simulink model "vehicle_model"  (R2023a)
settings: configuration reference "SharedConfig" (kept outside this file)
undefined symbols (not defined in the file): config_vehicle
settings Model: Creator=frede  LastModifiedBy=polashehata
settings ConfigSetRef: SourceName=SharedConfig  SourceLocation=Base Workspace

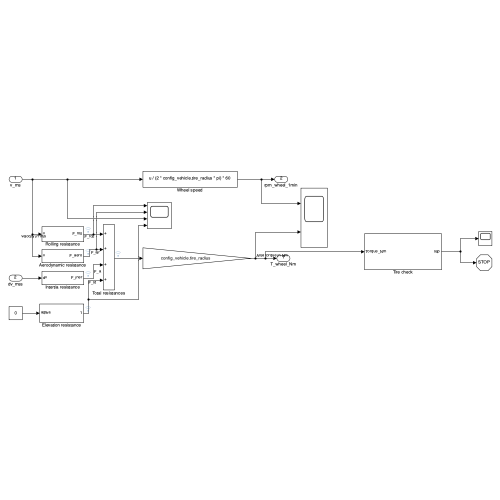
[thumbnail: Simulink's stored preview of the top-level diagram]
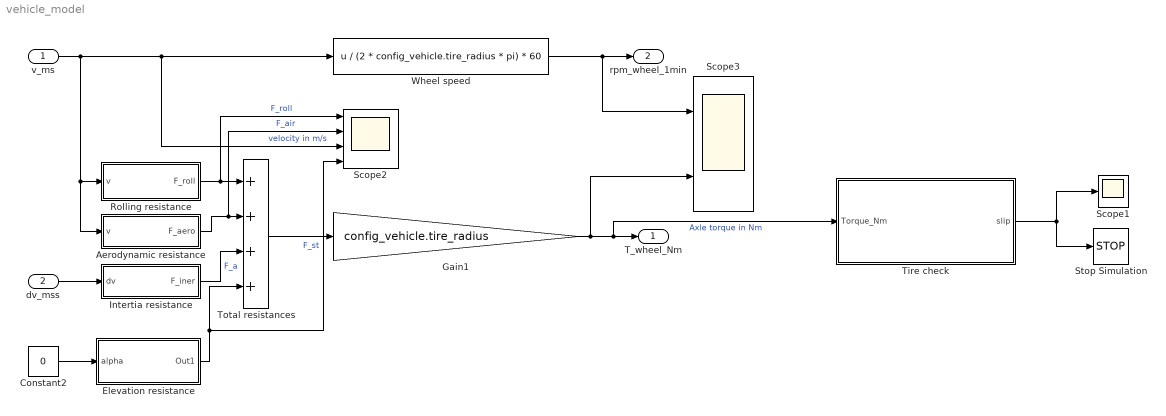
== system vehicle_model ==
  v_ms : Inport
  dv_mss : Inport  Port=2
  Aerodynamic resistance : Subsystem
  Constant2 : Constant  Value=0
  Elevation resistance : Subsystem
  Gain1 : Gain  Gain=config_vehicle.tire_radius
  Intertia resistance : Subsystem
  Rolling resistance : Subsystem
  Scope1 : Scope
  Scope2 : Scope  NumInputPorts=4
  Scope3 : Scope  NumInputPorts=2
  Stop Simulation : Stop
  Tire check : Subsystem
  Total resistances : Sum  Inputs=++++  InputSameDT=on  SaturateOnIntegerOverflow=on  OutDataTypeStr=Inherit: Same as first input
  Wheel speed : Fcn  Expr=u / (2 * config_vehicle.tire_radius * pi) * 60
  T_wheel_Nm : Outport  VectorParamsAs1DForOutWhenUnconnected=off
  rpm_wheel_1min : Outport  Port=2  VectorParamsAs1DForOutWhenUnconnected=off
  wires:
  dv_mss/1 -> Intertia resistance/1(dv)
  Wheel speed/1 -> rpm_wheel_1min/1, Scope3/1
  Aerodynamic resistance/1(F_aero) -> Scope2/2, Total resistances/2  "F_air"
  Intertia resistance/1(F_iner) -> Total resistances/3  "F_a"
  Gain1/1 -> Tire check/1(Torque_Nm), T_wheel_Nm/1, Scope3/2  "Axle torque in Nm"
  v_ms/1 -> Scope2/3, Wheel speed/1, Aerodynamic resistance/1(v), Rolling resistance/1(v)  "velocity in m/s"
  Rolling resistance/1(F_roll) -> Scope2/1, Total resistances/1  "F_roll"
  Tire check/1(slip) -> Scope1/1, Stop Simulation/1
  Constant2/1 -> Elevation resistance/1(alpha)
  Elevation resistance/1(Out1) -> Total resistances/4, Scope2/4  "F_st"
  Total resistances/1 -> Gain1/1

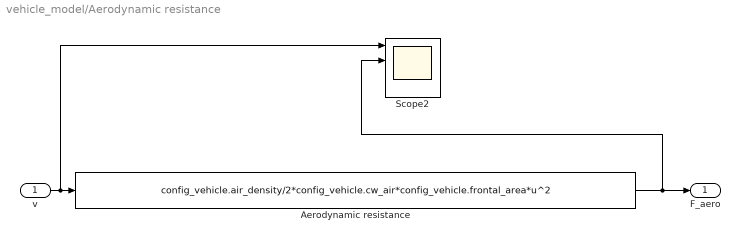
== system vehicle_model/Aerodynamic resistance ==
  v : Inport
  Aerodynamic resistance : Fcn  Expr=config_vehicle.air_density/2*config_vehicle.cw_air*config_vehicle.frontal_area*u^2
  Scope2 : Scope  NumInputPorts=4
  F_aero : Outport  VectorParamsAs1DForOutWhenUnconnected=off
  wires:
  Aerodynamic resistance/1 -> Scope2/2, F_aero/1
  v/1 -> Scope2/1, Aerodynamic resistance/1

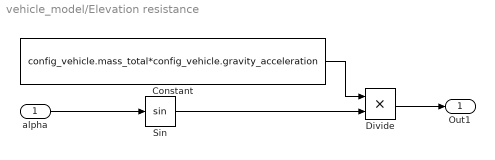
== system vehicle_model/Elevation resistance ==
  alpha : Inport
  Constant : Constant  Value=config_vehicle.mass_total*config_vehicle.gravity_acceleration
  Divide : Product  Inputs=**
  Sin : Trigonometry
  Out1 : Outport
  wires:
  Constant/1 -> Divide/1
  Divide/1 -> Out1/1
  alpha/1 -> Sin/1
  Sin/1 -> Divide/2

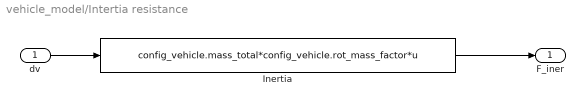
== system vehicle_model/Intertia resistance ==
  dv : Inport
  Inertia : Fcn  Expr=config_vehicle.mass_total*config_vehicle.rot_mass_factor*u
  F_iner : Outport  VectorParamsAs1DForOutWhenUnconnected=off
  wires:
  dv/1 -> Inertia/1
  Inertia/1 -> F_iner/1

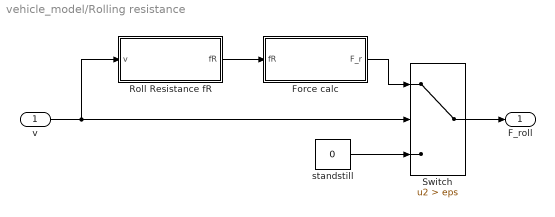
== system vehicle_model/Rolling resistance ==
  v : Inport
  Force calc : Subsystem
  Roll Resistance fR : Subsystem
  Switch : Switch  Criteria=u2 > Threshold  Threshold=eps  SaturateOnIntegerOverflow=off  InputSameDT=off
  standstill : Constant  Value=0
  F_roll : Outport  VectorParamsAs1DForOutWhenUnconnected=off
  wires:
  standstill/1 -> Switch/3
  Switch/1 -> F_roll/1
  v/1 -> Switch/2, Roll Resistance fR/1(v)
  Roll Resistance fR/1(fR) -> Force calc/1(fR)
  Force calc/1(F_r) -> Switch/1

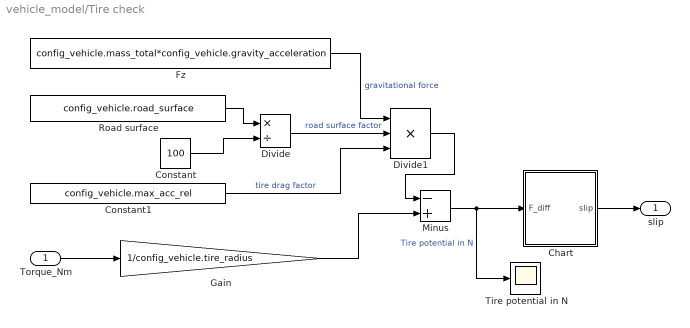
== system vehicle_model/Tire check ==
  Torque_Nm : Inport
  Chart : Stateflow chart  TreatAsAtomicUnit=on
  Constant : Constant  Value=100
  Constant1 : Constant  Value=config_vehicle.max_acc_rel
  Divide : Product  Inputs=*/  RndMeth=Zero  SaturateOnIntegerOverflow=on
  Divide1 : Product  Inputs=***  RndMeth=Zero  SaturateOnIntegerOverflow=on
  Fz : Constant  Value=config_vehicle.mass_total*config_vehicle.gravity_acceleration
  Gain : Gain  Gain=1/config_vehicle.tire_radius
  Minus : Sum  Inputs=-+
  Road surface : Constant  Value=config_vehicle.road_surface
  Tire potential in N : Scope
  slip : Outport
  wires:
  Road surface/1 -> Divide/1
  Constant/1 -> Divide/2
  Divide/1 -> Divide1/2  "road surface factor"
  Constant1/1 -> Divide1/3  "tire drag factor"
  Fz/1 -> Divide1/1  "gravitational force"
  Divide1/1 -> Minus/1
  Torque_Nm/1 -> Gain/1
  Gain/1 -> Minus/2
  Minus/1 -> Tire potential in N/1, Chart/1(F_diff)  "Tire potential in N"
  Chart/1(slip) -> slip/1

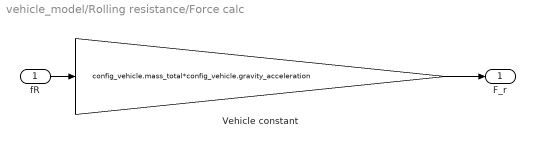
== system vehicle_model/Rolling resistance/Force calc ==
  fR : Inport
  Vehicle constant : Gain  Gain=config_vehicle.mass_total*config_vehicle.gravity_acceleration
  F_r : Outport
  wires:
  fR/1 -> Vehicle constant/1
  Vehicle constant/1 -> F_r/1

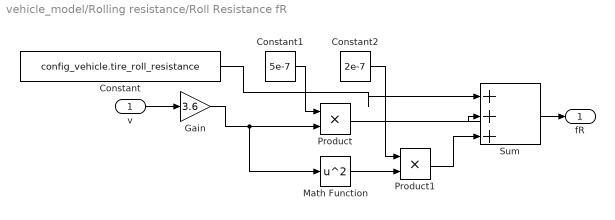
== system vehicle_model/Rolling resistance/Roll Resistance fR ==
  v : Inport
  Constant : Constant  Value=config_vehicle.tire_roll_resistance
  Constant1 : Constant  Value=5e-7
  Constant2 : Constant  Value=2e-7
  Gain : Gain  Gain=3.6
  Math Function : Math  Operator=square
  Product : Product
  Product1 : Product
  Sum : Sum  Inputs=|+++
  fR : Outport
  wires:
  Sum/1 -> fR/1
  Constant/1 -> Sum/1
  Constant1/1 -> Product/1
  Product/1 -> Sum/2
  v/1 -> Gain/1
  Constant2/1 -> Product1/1
  Product1/1 -> Sum/3
  Math Function/1 -> Product1/2
  Gain/1 -> Math Function/1, Product/2

== stateflow chart vehicle_model/Tire check/Chart ==
  (default) -> (junction 14) : % test
  (junction 14) -> (junction 15) [order 1] : [F_diff > 0]
  (junction 14) -> (junction 16) [order 2] : {slip=0;}
  (junction 15) -> (junction 17) : {disp('Slip detected! Change acc profile');
      | slip=1;}
  (junction 17) -> (junction 16)
  (junction 16) -> (junction 18)
  data: F_diff input; slip output
